simulink model "P5_RCAP"  (R2020b)
settings: Solver=VariableStepAuto  StartTime=0.0  StopTime=10.0  RelTol=1e-3
model workspace (MAT data in the model file):
  C = 10
  R = 10
settings Model: Creator=mluser  LastModifiedBy=mluser

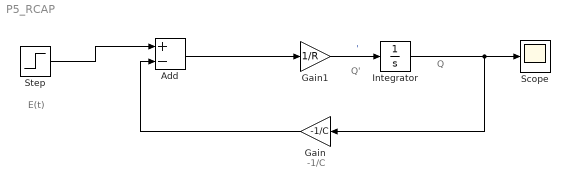
== system P5_RCAP ==
  note: -1/C
  note: E(t)
  note: Q'
  note: Q
  Add : Sum  Inputs=+-
  Gain : Gain  Gain=-1/C
  Gain1 : Gain  Gain=1/R
  Integrator : Integrator  InitialCondition=0.5
  Scope : Scope
  Step : Step  SampleTime=0
  wires:
  Add/1 -> Gain1/1
  Integrator/1 -> Scope/1, Gain/1
  Gain/1 -> Add/2
  Step/1 -> Add/1
  Gain1/1 -> Integrator/1  "'"
